simulink model "Exercise_3_Linear_Euler"  (R2021b)
settings: Solver=VariableStepAuto  StartTime=0.0  StopTime=simTime  FixedStep=0.001  RelTol=1e-3
undefined symbols (not defined in the file): AA, att_Kd, att_Ki, att_Kp, b, BB, CC, DD, g, k, L, m, MoI, posZ_Ki, posZ_Kp, RPM, TakeStep, Theta, uss, x0, xss
settings Model: Creator=Wojciech  LastModifiedBy=tanzc

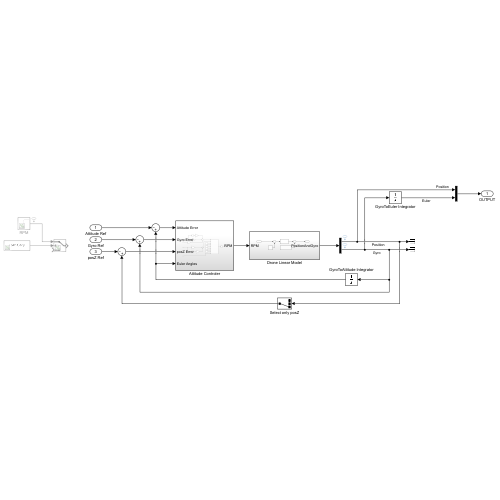
[thumbnail: Simulink's stored preview of the top-level diagram]
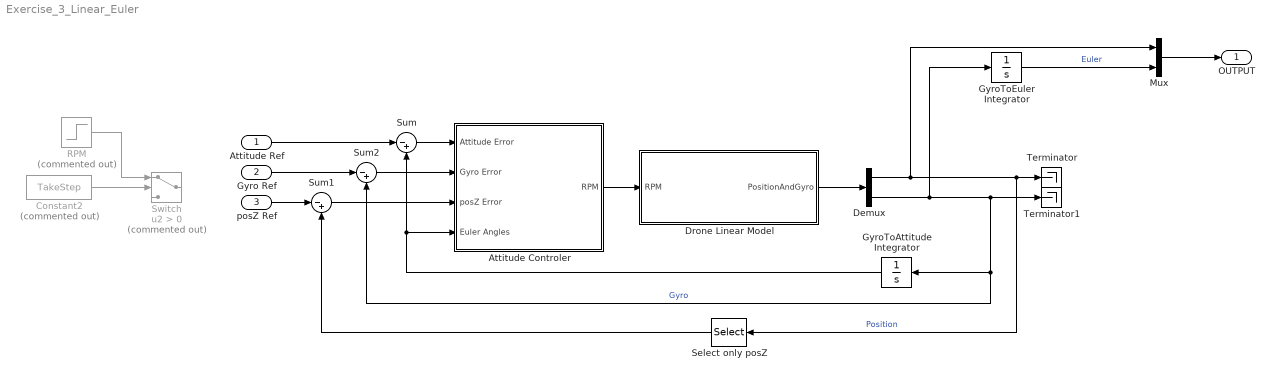
== system Exercise_3_Linear_Euler ==
  Attitude Ref : Inport  PortDimensions=3
  Gyro Ref : Inport  Port=2  PortDimensions=3
  posZ Ref : Inport  Port=3  PortDimensions=1
  Attitude Controler : Subsystem
  Constant2 : Constant  Commented=on  Value=TakeStep
  Demux : Demux  Outputs=2
  Drone Linear Model : Subsystem
  GyroToAttitude Integrator : Integrator  InitialCondition=Theta
  GyroToEuler Integrator : Integrator  InitialCondition=Theta
  Mux : Mux  Inputs=2
  RPM : Step  Commented=on  Time=0  After=RPM  SampleTime=0
  Select only posZ : Selector  InputPortWidth=3  IndexOptions=Index vector (dialog)  Indices=[3]  OutputSizes=1
  Sum : Sum  Inputs=|-+
  Sum1 : Sum  Inputs=|-+
  Sum2 : Sum  Inputs=|-+
  Switch : Switch  Commented=on  Criteria=u2 > Threshold
  Terminator : Terminator
  Terminator1 : Terminator
  OUTPUT : Outport
  wires:
  RPM/1 -> Switch/1
  Constant2/1 -> Switch/2
  Drone Linear Model/1(PositionAndGyro) -> Demux/1
  Demux/1 -> Mux/1, Select only posZ/1, Terminator/1  "Position"
  Demux/2 -> GyroToEuler Integrator/1, Sum2/2, GyroToAttitude Integrator/1, Terminator1/1  "Gyro"
  Attitude Ref/1 -> Sum/1
  posZ Ref/1 -> Sum1/1
  Select only posZ/1 -> Sum1/2
  Attitude Controler/1(RPM) -> Drone Linear Model/1(RPM)
  Sum/1 -> Attitude Controler/1(Attitude Error)
  Sum1/1 -> Attitude Controler/3(posZ Error)
  GyroToEuler Integrator/1 -> Mux/2  "Euler"
  Mux/1 -> OUTPUT/1
  Sum2/1 -> Attitude Controler/2(Gyro Error)
  Gyro Ref/1 -> Sum2/1
  GyroToAttitude Integrator/1 -> Sum/2, Attitude Controler/4(Euler Angles)

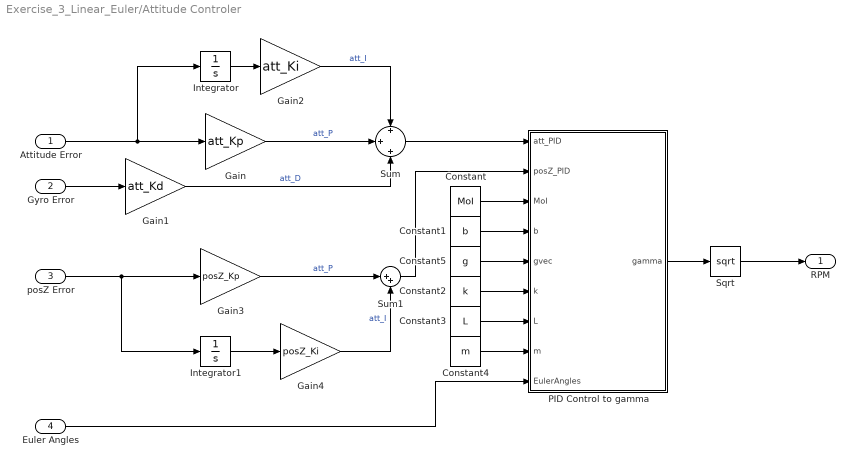
== system Exercise_3_Linear_Euler/Attitude Controler ==
  Attitude Error : Inport
  Gyro Error : Inport  Port=2
  posZ Error : Inport  Port=3
  Euler Angles : Inport  Port=4
  Constant : Constant  Value=MoI
  Constant1 : Constant  Value=b
  Constant2 : Constant  Value=k
  Constant3 : Constant  Value=L
  Constant4 : Constant  Value=m
  Constant5 : Constant  Value=g
  Gain : Gain  Gain=att_Kp
  Gain1 : Gain  Gain=att_Kd
  Gain2 : Gain  Gain=att_Ki
  Gain3 : Gain  Gain=posZ_Kp
  Gain4 : Gain  Gain=posZ_Ki
  Integrator : Integrator  Priority=1  InitialCondition=[0, 0, 0]'
  Integrator1 : Integrator  Priority=2
  PID Control to gamma : MATLAB Function  TreatAsAtomicUnit=on
  Sqrt : Sqrt  SaturateOnIntegerOverflow=on
  Sum : Sum  Inputs=+|+|+
  Sum1 : Sum  Inputs=|++
  RPM : Outport
  wires:
  Attitude Error/1 -> Gain/1, Integrator/1
  Gyro Error/1 -> Gain1/1
  Integrator/1 -> Gain2/1
  Gain/1 -> Sum/2  "att_P"
  Gain2/1 -> Sum/1  "att_I"
  Gain1/1 -> Sum/3  "att_D"
  posZ Error/1 -> Integrator1/1, Gain3/1
  Integrator1/1 -> Gain4/1
  Gain3/1 -> Sum1/1  "att_P"
  Gain4/1 -> Sum1/2  "att_I"
  Sum/1 -> PID Control to gamma/1(att_PID)
  Sum1/1 -> PID Control to gamma/2(posZ_PID)
  Constant/1 -> PID Control to gamma/3(MoI)
  Constant1/1 -> PID Control to gamma/4(b)
  Constant2/1 -> PID Control to gamma/6(k)
  Constant3/1 -> PID Control to gamma/7(L)
  Euler Angles/1 -> PID Control to gamma/9(EulerAngles)
  Constant4/1 -> PID Control to gamma/8(m)
  Constant5/1 -> PID Control to gamma/5(gvec)
  PID Control to gamma/1(gamma) -> Sqrt/1
  Sqrt/1 -> RPM/1

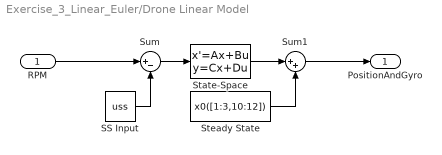
== system Exercise_3_Linear_Euler/Drone Linear Model ==
  RPM : Inport
  SS Input : Constant  Value=uss  VectorParams1D=off
  State-Space : StateSpace  A=AA  B=BB  C=CC  D=DD  InitialCondition=xss
  Steady State : Constant  Value=x0([1:3,10:12])  VectorParams1D=off
  Sum : Sum  Inputs=|+-
  Sum1 : Sum  Inputs=|++
  PositionAndGyro : Outport
  wires:
  State-Space/1 -> Sum1/1
  Steady State/1 -> Sum1/2
  SS Input/1 -> Sum/2
  Sum/1 -> State-Space/1
  Sum1/1 -> PositionAndGyro/1
  RPM/1 -> Sum/1

== matlab function Exercise_3_Linear_Euler/Attitude Controler/PID Control to gamma ==
  data: att_PID input; gamma output; posZ_PID input; MoI input; b input; gvec input; k input; L input; m input; EulerAngles input
function gamma = fcn(att_PID, posZ_PID, MoI, b, gvec, k, L, m, EulerAngles)

u_phi   = att_PID(1);
u_theta = att_PID(2);
u_psi   = att_PID(3);

u_posZ = posZ_PID;

Ixx = MoI(1,1);
Iyy = MoI(2,2);
Izz = MoI(3,3);

g = -gvec(3);

phi     = EulerAngles(1); 
theta   = EulerAngles(2);
psi     = EulerAngles(3);

gamma1 = m*(g + u_posZ)/(4*k*cos(theta)*cos(phi)) - (2*b*u_phi*Ixx + u_psi*Izz*k*L)/(4*b*k*L);
gamma2 = m*(g + u_posZ)/(4*k*cos(theta)*cos(phi)) + u_psi*Izz/4/b - u_theta*Iyy/2/k/L;
gamma3 = m*(g + u_posZ)/(4*k*cos(theta)*cos(phi)) - (-2*b*u_phi*Ixx + u_psi*Izz*k*L)/(4*b*k*L);
gamma4 = m*(g + u_posZ)/(4*k*cos(theta)*cos(phi)) + u_psi*Izz/4/b + u_theta*Iyy/2/k/L;

gamma = [gamma1, gamma2, gamma3, gamma4]';
